simulink model "model2_control"  (R2025b)
settings: Solver=ode45  StartTime=0.0  StopTime=10  MaxStep=0.00012566370614359171  RelTol=1e-7  AbsTol=1e-9
values from neighbouring files (symbols this model uses):
  p = [g; L; zeta; A; f]    [kapitza_controle.m]    (also in parameters_kapitza_model2.m)
  pc = [c1; c2; alpha_ctrl]    [kapitza_controle.m]
  x0 = [150*pi/180; 0]    [kapitza_controle.m]    (also in parameters_kapitza_model2.m = [45*pi/180; 0])
libraries: simulink x1
settings Model: Creator=rafae  LastModifiedBy=rafae
settings SolverCC: AutoScaleAbsTol=off

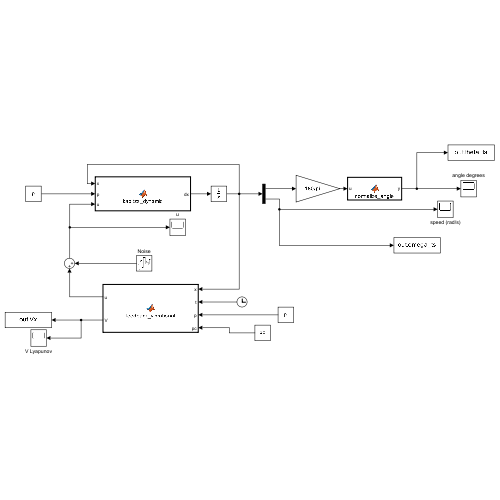
[thumbnail: Simulink's stored preview of the top-level diagram]
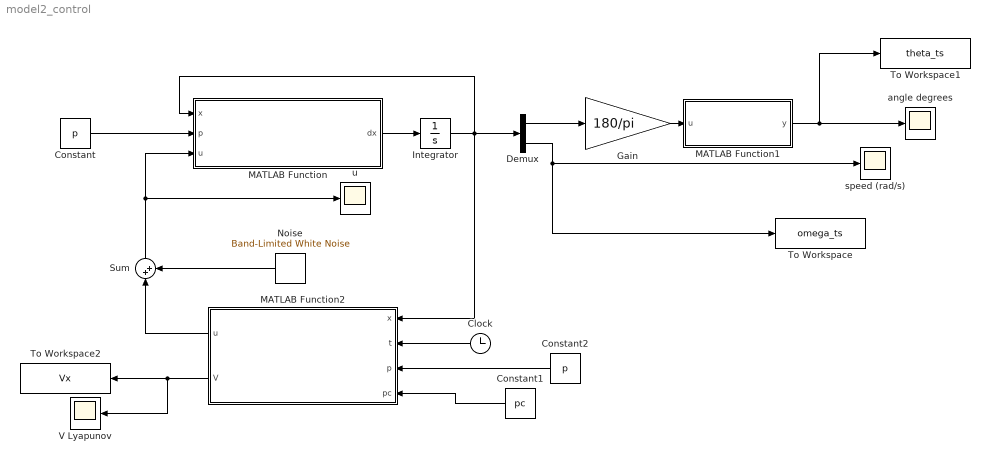
== system model2_control ==
  Clock : Clock
  Constant : Constant  Value=p
  Constant1 : Constant  Value=pc
  Constant2 : Constant  Value=p
  Demux : Demux  Outputs=2
  Gain : Gain  Gain=180/pi
  Integrator : Integrator  InitialCondition=x0
  MATLAB Function : MATLAB Function  TreatAsAtomicUnit=on
  MATLAB Function1 : MATLAB Function  TreatAsAtomicUnit=on
  MATLAB Function2 : MATLAB Function  TreatAsAtomicUnit=on
  Noise : simulink/Sources/Band-Limited White Noise  Cov=[5]  Ts=0.1  seed=[23341]
  Sum : Sum  Inputs=|++
  To Workspace : ToWorkspace  VariableName=omega_ts  SaveFormat=Timeseries  SampleTime=-1
  To Workspace1 : ToWorkspace  VariableName=theta_ts  SaveFormat=Timeseries  SampleTime=-1
  To Workspace2 : ToWorkspace  VariableName=Vx  SaveFormat=Timeseries  SampleTime=-1
  V Lyapunov : Scope
      settings: ActiveDisplayYMinimum=-19.231103634644647  ActiveDisplayYMaximum=173.079932712719  DataLoggingVariableName=ScopeData2
  angle degrees : Scope
      settings: ActiveDisplayYMinimum=-22.674305632538491  ActiveDisplayYMaximum=152.63845772950825
  speed (rad/s) : Scope
      settings: ActiveDisplayYMinimum=-1  ActiveDisplayYMaximum=1
  u : Scope
      settings: ActiveDisplayYMinimum=-2266.8538508977153  ActiveDisplayYMaximum=2257.9626335766143  DataLoggingVariableName=ScopeData3
  wires:
  Clock/1 -> MATLAB Function2/2(t)
  Constant/1 -> MATLAB Function/2(p)
  MATLAB Function/1(dx) -> Integrator/1
  Integrator/1 -> MATLAB Function2/1(x), MATLAB Function/1(x), Demux/1
  Demux/2 -> speed (rad/s)/1, To Workspace/1
  Gain/1 -> MATLAB Function1/1(u)
  Demux/1 -> Gain/1
  MATLAB Function1/1(y) -> To Workspace1/1, angle degrees/1
  Constant1/1 -> MATLAB Function2/4(pc)
  MATLAB Function2/2(V) -> V Lyapunov/1, To Workspace2/1
  MATLAB Function2/1(u) -> Sum/1
  Sum/1 -> MATLAB Function/3(u), u/1
  Noise/1 -> Sum/2
  Constant2/1 -> MATLAB Function2/3(p)

== matlab function model2_control/MATLAB Function1 ==
  data: u input; y output
function y = normalize_angle(u)
    y = mod(u + 180, 360) - 180;
end

== matlab function model2_control/MATLAB Function ==
  data: x input; dx output; p input; u input
function dx = kapitza_dynamic(x, p, u)%#codegen

g = p(1);
L = p(2);
zeta = p(3);

theta = x(1);
velocidade = x(2);

wn = sqrt(g/L);

dx = zeros(2,1);
dx(1) = velocidade;

dx(2) = -2*zeta*wn*velocidade ...
        + (g/L-u/L)*sin(theta);
end

== matlab function model2_control/MATLAB Function2 ==
  data: x input; u output; t input; p input; pc input; V output
function [u, V] = feedback_vibrational(x, t, p, pc)
%#codegen

A = p(4);
f = p(5);

c1 = pc(1);
c2 = pc(2);

theta = x(1);
velocidade = x(2);

w = 2*pi*f;

V1 = c1*(1 - cos(theta));
V2 = 0.5*(c2*velocidade + sin(theta))^2;
V  = V1 + V2;

u = A*w^2*cos(w*t) - sqrt(w)*V*sin(w*t);

end
